simulink model "A34hij"  (R2022b)
settings: Solver=VariableStepAuto  StartTime=0.0  StopTime=80  RelTol=1e-3
values from neighbouring files (symbols this model uses):
  ainv = [1 0 0 0.8]    [a34abcd.m]    (also in a34efg.m = [hk])
  bapp = [1 0 0 -0.8 0 0 0.64 0 0 -0.512]    [a34abcd.m]    (also in a34efg.m = [happ])
  binv = [1]    [a34abcd.m]    (also in a34efg.m)
libraries: commrandsrc3 x1, dspsigops x1
settings Model: Creator=Feldes  LastModifiedBy=Labor
settings DebuggingCC: UnconnectedInputMsg=warning  UnconnectedOutputMsg=warning  UnconnectedLineMsg=warning
settings ModelReferenceCC: EnableRefExpFcnMdlSchedulingChecks=on
settings RTWCC: DLArmComputeVersion=19.05

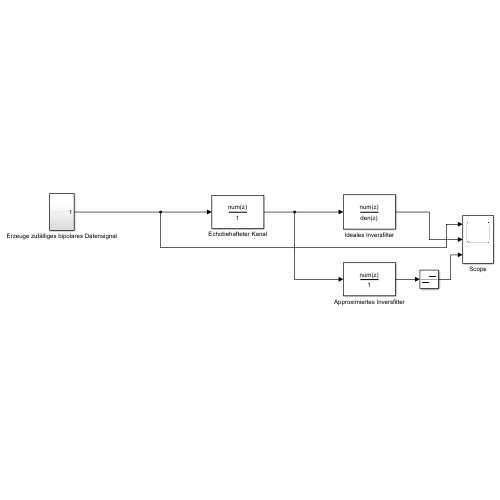
[thumbnail: Simulink's stored preview of the top-level diagram]
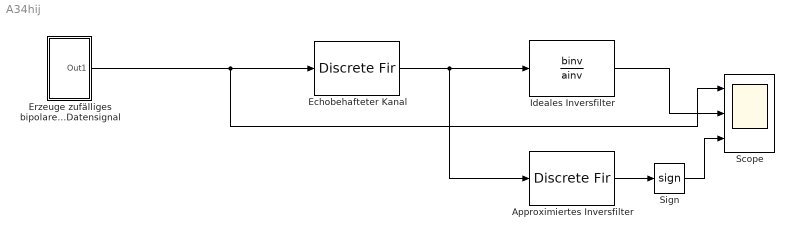
== system A34hij ==
  Approximiertes Inversfilter : DiscreteFir  Coefficients=bapp  InputProcessing=Columns as channels (frame based)
  Echobehafteter Kanal : DiscreteFir  Coefficients=[1 zeros(1,7) 0.6 zeros(1,4) 0.4]
  Erzeuge zufälliges bipolares Datensignal : Subsystem
  Ideales Inversfilter : DiscreteFilter  Numerator=binv  Denominator=ainv  InputProcessing=Columns as channels (frame based)  FilterStructure=Direct form II transposed  a0EqualsOne=on
  Scope : Scope  NumInputPorts=3
  Sign : Signum
  wires:
  Approximiertes Inversfilter/1 -> Sign/1
  Erzeuge zufälliges bipolares Datensignal/1(Out1) -> Scope/1, Echobehafteter Kanal/1
  Echobehafteter Kanal/1 -> Approximiertes Inversfilter/1, Ideales Inversfilter/1
  Sign/1 -> Scope/3
  Ideales Inversfilter/1 -> Scope/2

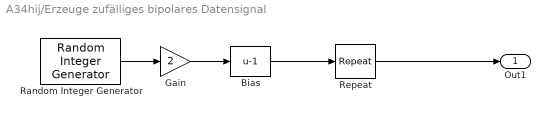
== system A34hij/Erzeuge zufälliges bipolares Datensignal ==
  Bias : Bias  Bias=-1  SaturateOnIntegerOverflow=off
  Gain : Gain  Gain=2
  Random Integer Generator : commrandsrc3/Random Integer Generator  SetSize=2  SeedSource=Parameter  Seed=120  SampleTime=1  SamplesPerFrame=1  OutputDataType=double  SimulateUsing=Interpreted execution
  Repeat : dspsigops/Repeat  N=10  RateOptions=Allow multirate processing  ic=0  mode=Unused parameter value
  Out1 : Outport
  wires:
  Gain/1 -> Bias/1
  Random Integer Generator/1 -> Gain/1
  Bias/1 -> Repeat/1
  Repeat/1 -> Out1/1
